simulink model "RTPS_2018a"  (R2018a)
settings: Solver=FixedStepAuto  StartTime=0.0  StopTime=150  RelTol=1e-3
settings Model: Creator=root  LastModifiedBy=bzhan
settings RTWCC: Description=Create Visual C/C++ Solution File for Simulink Coder  TemplateMakefile=RTW.MSVCBuild
settings CodeAppCC: StateflowObjectComments=on

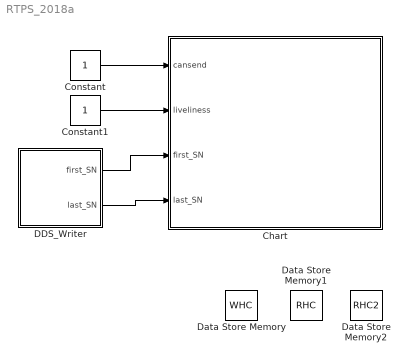
== system RTPS_2018a ==
  Chart : Stateflow chart  TreatAsAtomicUnit=on
  Constant : Constant
  Constant1 : Constant
  DDS_Writer : Stateflow chart  TreatAsAtomicUnit=on
  Data Store Memory : DataStoreMemory  DataStoreName=WHC  ReadBeforeWriteMsg=warning  WriteAfterWriteMsg=warning  WriteAfterReadMsg=warning  InitialValue=[0 0 0 0 0]  ShowAdditionalParam=off  OutDataTypeStr=int32
  Data Store Memory1 : DataStoreMemory  DataStoreName=RHC  ReadBeforeWriteMsg=warning  WriteAfterWriteMsg=warning  WriteAfterReadMsg=warning  InitialValue=[0 0 0 0 0]  VectorParams1D=off  ShowAdditionalParam=off  OutDataTypeStr=int32
  Data Store Memory2 : DataStoreMemory  DataStoreName=RHC2  ReadBeforeWriteMsg=warning  WriteAfterWriteMsg=warning  WriteAfterReadMsg=warning  InitialValue=[0 0 0 0 0]  VectorParams1D=off  ShowAdditionalParam=off  OutDataTypeStr=int32
  wires:
  Constant/1 -> Chart/1(cansend)
  Constant1/1 -> Chart/2(liveliness)
  DDS_Writer/1(first_SN) -> Chart/3(first_SN)
  DDS_Writer/2(last_SN) -> Chart/4(last_SN)

== stateflow chart RTPS_2018a/DDS_Writer ==
  state add
  (default) -> add : {i=1;first_SN=1;last_SN=0;d=random()}
  add -> add : after(d,sec)[i<=5]
      | {WHC(i)=cachechanges(i);
      | first_SN=1;last_SN=i;i = i + 1;d=random()}
  data: y function_output; i local; first_SN output; last_SN output; WHC data_store_memory; flag local; cachechanges local =[100,200,300,400,500]; d local
  function y=random:
    | function y=random
    |   y=rand();

== stateflow chart RTPS_2018a/Chart ==
  state select_channel(i) [function]
    (junction 462) -> (junction 468) [order 1] : [i==1]
    (junction 468) -> (junction 471) : {send(TRY,model.channel.channel_1)}
    (junction 462) -> (junction 466) [order 2] : [i==2]
    (junction 466) -> (junction 471) : {send(TRY,model.channel.channel_2)}
    (default) -> (junction 462)
    (junction 462) -> (junction 465) [order 3] : [i==3]
    (junction 465) -> (junction 471) : {send(TRY,model.channel.channel_3)}
    (junction 462) -> (junction 464) [order 4] : [i==4]
    (junction 462) -> (junction 463) [order 5]
    (junction 464) -> (junction 471) : {send(TRY,model.channel.channel_4)}
    (junction 463) -> (junction 471) : {send(TRY,model.channel.channel_5)}
  state set_acknack(wid,rid,rn,mn) [function]
    (default) -> (junction 110)
    (junction 110) -> (junction 103) : {buffer_acknack(rid,1)=1;
        | buffer_acknack(rid,2)=rid}
    (junction 103) -> (junction 104) : {buffer_acknack(rid,3)=rn;
        | buffer_acknack(rid,4)=mn}
  state flag=acked_all [function]
    (junction 625) -> (junction 624) [order 3]
    (junction 624) -> (junction 627) : {flag=0}
    (default) -> (junction 625) : {i=1}
    (junction 625) -> (junction 626) [order 1] : [i>2]
    (junction 626) -> (junction 627) : {flag=1}
    (junction 627) -> (junction 628)
    (junction 630) -> (junction 625)
    (junction 625) -> (junction 631) [order 2] : [i<=2&&buffer_acknack(i,3)==5]
    (junction 631) -> (junction 630) : {i = i + 1}
  state flag=empty [function]
    (junction 11) -> (junction 10) [order 3]
    (junction 10) -> (junction 13) : {flag=0}
    (default) -> (junction 11) : {i=first_SN}
    (junction 11) -> (junction 12) [order 1] : [i>last_SN]
    (junction 12) -> (junction 13) : {flag=1}
    (junction 13) -> (junction 14)
    (junction 16) -> (junction 11)
    (junction 11) -> (junction 18) [order 2] : [i<=last_SN&&unsent(i)==0]
    (junction 18) -> (junction 16) : {i = i + 1}
  state count1 = set_final_Flag(wid,count) [function]
    (junction 33) -> (junction 34) [order 2] : {buffer_heartbeat(wid,1)=SET;count1 = count + 1}
    (junction 34) -> (junction 35)
    (default) -> (junction 33)
    (junction 33) -> (junction 36) [order 1] : [count==3]
    (junction 37) -> (junction 34)
    (junction 36) -> (junction 37) : {buffer_heartbeat(wid,1)=NO_SET;count1=0}
  state set_liveliness_Flag(wid, flag) [function]
    (default) -> (junction 27)
    (junction 27) -> (junction 48) : {buffer_heartbeat(wid,2)=flag;}
  state set_heartbeatSN(wid) [function]
    (default) -> (junction 79)
    (junction 79) -> (junction 80) : {buffer_heartbeat(wid,3)=first_SN}
    (junction 80) -> (junction 81) : {buffer_heartbeat(wid,4)=last_SN}
  state set_message(sn) [function]
    (junction 606) -> (junction 83) : {buffer_data(WriterId,i,sn)=WHC(sn);i = i + 1}
    (junction 83) -> (junction 47)
    (junction 47) -> (junction 606) [order 1] : [i<=2]
    (default) -> (junction 47) : {i=1}
    (junction 47) -> (junction 611) [order 2]
  state model
    state RTPS_Reader [parallel]
      settings: executionOrder=2
      state RTPS_Reader_2 [parallel]
        settings: executionOrder=2
        state Reader_receive [parallel]
          settings: executionOrder=1
          state ready
          model.RTPS_Reader.RTPS_Reader_2.Reader_receive.ready -> model.RTPS_Reader.RTPS_Reader_2.Reader_receive.ready [order 2] : SUCCESS[seq_num_2>received_num2]
              | {index2=seq_num_2;
              | received_set(ReaderId_2,index2)=true;
              | received_num2=check_received(WriterId,ReaderId_2,received_num2);
              | missing_num2=check_missing(WriterId,ReaderId_2,missing_num2);
              | RHC2(index2)=buffer_data(WriterId,ReaderId_2,index2);
              | buffer_data(WriterId,ReaderId_2,index2)=false}
          model.RTPS_Reader.RTPS_Reader_2.Reader_receive.ready -> model.RTPS_Reader.RTPS_Reader_2.Reader_receive.ready [order 1] : HEARTBEAT2
              | {missing_num2=get_heartbeatSN(1,2);}
          (default) -> model.RTPS_Reader.RTPS_Reader_2.Reader_receive.ready
        state Reader_response [parallel]
          settings: executionOrder=2
          state must_send_ack
          state may_send_ack
          state waiting
          model.RTPS_Reader.RTPS_Reader_2.Reader_response.must_send_ack -> model.RTPS_Reader.RTPS_Reader_2.Reader_response.waiting : after(nackResponseDelay,sec)
              | {ack_id=ReaderId_2;
              | set_acknack(WriterId,ack_id,received_num2,missing_num2);
              | send(ACKNACK,model.channel_Acknack_2);
              | hFlag=0}
          model.RTPS_Reader.RTPS_Reader_2.Reader_response.may_send_ack -> model.RTPS_Reader.RTPS_Reader_2.Reader_response.must_send_ack [order 1] : [missing_num2>received_num2]
          (junction 191) -> model.RTPS_Reader.RTPS_Reader_2.Reader_response.must_send_ack [order 1] : [buffer_heartbeat(WriterId, livelinessFlag)==NO_SET]
          model.RTPS_Reader.RTPS_Reader_2.Reader_response.waiting -> (junction 191) : HEARTBEAT2{hFlag=1}
          (default) -> model.RTPS_Reader.RTPS_Reader_2.Reader_response.waiting
          (junction 191) -> model.RTPS_Reader.RTPS_Reader_2.Reader_response.may_send_ack [order 3]
          (junction 191) -> model.RTPS_Reader.RTPS_Reader_2.Reader_response.waiting [order 2] : [buffer_heartbeat(WriterId, finalFlag)==SET]{hFlag=0}
          model.RTPS_Reader.RTPS_Reader_2.Reader_response.may_send_ack -> model.RTPS_Reader.RTPS_Reader_2.Reader_response.waiting [order 2] : [missing_num2<=received_num2]{hFlag=0}
      state RTPS_Reader_1 [parallel]
        settings: executionOrder=1
        state Reader_receive [parallel]
          settings: executionOrder=1
          state ready
          model.RTPS_Reader.RTPS_Reader_1.Reader_receive.ready -> model.RTPS_Reader.RTPS_Reader_1.Reader_receive.ready [order 2] : SUCCESS[seq_num_1>received_num]
              | {index=seq_num_1;received_set(WriterId,index)=true;
              | received_num=check_received(WriterId,ReaderId_1,received_num);
              | missing_num=check_missing(WriterId,ReaderId_1,missing_num);
              | RHC(index)=buffer_data(WriterId,ReaderId_1,index);
              | buffer_data(WriterId,ReaderId_1,index)=false;}
          (default) -> model.RTPS_Reader.RTPS_Reader_1.Reader_receive.ready
          model.RTPS_Reader.RTPS_Reader_1.Reader_receive.ready -> model.RTPS_Reader.RTPS_Reader_1.Reader_receive.ready [order 1] : HEARTBEAT2
              | {missing_num=get_heartbeatSN(1,1);}
        state Reader_response [parallel]
          settings: executionOrder=2
          state must_send_ack
          state waiting
          state may_send_ack
          model.RTPS_Reader.RTPS_Reader_1.Reader_response.must_send_ack -> model.RTPS_Reader.RTPS_Reader_1.Reader_response.waiting : after(nackResponseDelay,sec)
              | {ack_id=ReaderId_1;
              | set_acknack(WriterId,ack_id,received_num,missing_num);
              | send(ACKNACK,model.channel_Acknack_1);
              | hFlag=0}
          model.RTPS_Reader.RTPS_Reader_1.Reader_response.may_send_ack -> model.RTPS_Reader.RTPS_Reader_1.Reader_response.must_send_ack [order 1] : [missing_num>received_num]
          (junction 224) -> model.RTPS_Reader.RTPS_Reader_1.Reader_response.must_send_ack [order 1] : [buffer_heartbeat(WriterId, livelinessFlag)==NO_SET]
          model.RTPS_Reader.RTPS_Reader_1.Reader_response.waiting -> (junction 224) : HEARTBEAT2{hFlag=1}
          (junction 224) -> model.RTPS_Reader.RTPS_Reader_1.Reader_response.may_send_ack [order 3]
          (junction 224) -> model.RTPS_Reader.RTPS_Reader_1.Reader_response.waiting [order 2] : [buffer_heartbeat(WriterId, finalFlag)==SET]
              | {hFlag=0}
          (default) -> model.RTPS_Reader.RTPS_Reader_1.Reader_response.waiting
          model.RTPS_Reader.RTPS_Reader_1.Reader_response.may_send_ack -> model.RTPS_Reader.RTPS_Reader_1.Reader_response.waiting [order 2] : [missing_num<=received_num]{hFlag=0}
    state RTPS_Writer [parallel]
      settings: executionOrder=1
      state Writer_send [parallel]
        settings: executionOrder=2
        state pushing
        state announcing
        state idle
        announcing -> (junction 771) [order 1] : after(heartbeatPeriod,sec)
            | [acked_all()==false&&empty()==true]
            | {hb_count=set_final_Flag(WriterId,hb_count);
            | set_liveliness_Flag(WriterId, liveliness);
            | set_heartbeatSN(WriterId);
            | send(HEARTBEAT,model.channel_Heartbeat);
            |  sendFlag=1}
        (junction 771) -> announcing : {sendFlag=0}
        pushing -> pushing [order 2] : [cansend==true&&empty()==false]
            | {set_message(index);
            | select_channel(index);
            | unsent(index) = false;
            | index = index + 1}
        idle -> announcing : [acked_all()==false]
        announcing -> pushing [order 2] : [acked_all()==false&&empty()==false]
        announcing -> idle [order 3] : [acked_all()==true]{complete=true}
        pushing -> announcing [order 1] : [empty()==true]
        (default) -> announcing : {init()}
      state Writer_repair [parallel]
        settings: executionOrder=1
        state repairing
        state waiting
        state must_repair
          state en
          (default) -> en : {ackFlag=0}
          en -> en : ACKNACK2{id=ack_id;
              |  [acked_num(id),request_num(id)]=get_acknack(WriterId,id);
              | ackFlag=1}
        repairing -> repairing [order 1] : [cansend==true&&repair_num(id)<=request_num(id)]
            | {set_message(repair_num(id));
            | select_channel(repair_num(id));
            | repair_num(id) = repair_num(id) + 1}
        must_repair -> repairing : after(heartbeatResponseDelay,sec)
            | {repair_num(id)=acked_num(id)+1;
            | ackFlag=0}
        repairing -> model.RTPS_Writer.Writer_repair.waiting [order 2] : [cansend==false||repair_num(id)>request_num(id)]
        model.RTPS_Writer.Writer_repair.waiting -> must_repair [order 1] : [id>0&&request_num(id)>acked_num(id)]
        (default) -> model.RTPS_Writer.Writer_repair.waiting
        model.RTPS_Writer.Writer_repair.waiting -> model.RTPS_Writer.Writer_repair.waiting [order 2] : ACKNACK2
            | [id<=0||request_num(id)<=acked_num(id)]
            | {id=ack_id;
            | [acked_num(id),request_num(id)]=get_acknack(WriterId,id);
            | ackFlag=1}
    state channel_Heartbeat [parallel]
      settings: executionOrder=4
      state try
      state delay
      (default) -> model.channel_Heartbeat.try
      (junction 764) -> model.channel_Heartbeat.try [order 2]
      model.channel_Heartbeat.try -> (junction 764) : HEARTBEAT
      model.channel_Heartbeat.delay -> model.channel_Heartbeat.try : after(d_hb,sec)
          | {send(HEARTBEAT2,model.RTPS_Reader)}
      (junction 764) -> model.channel_Heartbeat.delay [order 1] : [channel()==true]{d_hb=delay()}
    state channel_Acknack_1 [parallel]
      settings: executionOrder=5
      state try
      state delay
      (default) -> model.channel_Acknack_1.try
      (junction 723) -> model.channel_Acknack_1.try [order 2]
      model.channel_Acknack_1.try -> (junction 723) : ACKNACK
      model.channel_Acknack_1.delay -> model.channel_Acknack_1.try : after(d_ack1,sec)
          | {ack_id=ReaderId_1;
          | send(ACKNACK2,model.RTPS_Writer)}
      (junction 723) -> model.channel_Acknack_1.delay [order 1] : [channel()==true]{d_ack1=delay()}
    state channel [parallel]
      settings: executionOrder=3
      state channel_4 [parallel]
        settings: executionOrder=4
        state try
        state delay_1
        state delay_2
        state next
        (default) -> model.channel.channel_4.try
        model.channel.channel_4.next -> model.channel.channel_4.try [order 2] : {buffer_data(WriterId,2,4)=0}
        model.channel.channel_4.try -> (junction 553) : TRY
        model.channel.channel_4.delay_2 -> model.channel.channel_4.try : after(d4,sec)
            | {seq_num_2=4;
            | send(SUCCESS,model.RTPS_Reader.RTPS_Reader_2)}
        (junction 553) -> model.channel.channel_4.delay_1 [order 1] : [channel()==true]{d4=delay()}
        (junction 553) -> model.channel.channel_4.next [order 2] : {buffer_data(WriterId,1,4)=0}
        model.channel.channel_4.delay_1 -> model.channel.channel_4.next : after(d4,sec)
            | {seq_num_1=4;
            | send(SUCCESS,model.RTPS_Reader.RTPS_Reader_1)}
        model.channel.channel_4.next -> model.channel.channel_4.delay_2 [order 1] : [channel()==true]{d4=delay()}
      state channel_5 [parallel]
        settings: executionOrder=5
        state try
        state delay_1
        state delay_2
        state next
        (default) -> model.channel.channel_5.try
        model.channel.channel_5.next -> model.channel.channel_5.try [order 2] : {buffer_data(WriterId,2,5)=0}
        model.channel.channel_5.try -> (junction 571) : TRY
        model.channel.channel_5.delay_2 -> model.channel.channel_5.try : after(d5,sec)
            | {seq_num_2=5;
            | send(SUCCESS,model.RTPS_Reader.RTPS_Reader_2)}
        (junction 571) -> model.channel.channel_5.delay_1 [order 1] : [channel()==true]{d5=delay()}
        (junction 571) -> model.channel.channel_5.next [order 2] : {buffer_data(WriterId,1,5)=0}
        model.channel.channel_5.delay_1 -> model.channel.channel_5.next : after(d5,sec)
            | {seq_num_1=5;
            | send(SUCCESS,model.RTPS_Reader.RTPS_Reader_1)}
        model.channel.channel_5.next -> model.channel.channel_5.delay_2 [order 1] : [channel()==true]{d5=delay()}
      state channel_2 [parallel]
        settings: executionOrder=2
        state try
        state delay_1
        state delay_2
        state next
        (default) -> model.channel.channel_2.try
        model.channel.channel_2.next -> model.channel.channel_2.try [order 2] : {buffer_data(WriterId,2,2)=0}
        model.channel.channel_2.try -> (junction 517) : TRY
        model.channel.channel_2.delay_2 -> model.channel.channel_2.try : after(d2,sec)
            | {seq_num_2=2;
            | send(SUCCESS,model.RTPS_Reader.RTPS_Reader_2)}
        (junction 517) -> model.channel.channel_2.delay_1 [order 1] : [channel()==true]{d2=delay()}
        (junction 517) -> model.channel.channel_2.next [order 2] : {buffer_data(WriterId,1,2)=0}
        model.channel.channel_2.delay_1 -> model.channel.channel_2.next : after(d2,sec)
            | {seq_num_1=2;
            | send(SUCCESS,model.RTPS_Reader.RTPS_Reader_1)}
        model.channel.channel_2.next -> model.channel.channel_2.delay_2 [order 1] : [channel()==true]{d2=delay()}
      state channel_3 [parallel]
        settings: executionOrder=3
        state try
        state delay_1
        state delay_2
        state next
        (default) -> model.channel.channel_3.try
        model.channel.channel_3.next -> model.channel.channel_3.try [order 2] : {buffer_data(WriterId,2,3)=0}
        model.channel.channel_3.try -> (junction 535) : TRY
        model.channel.channel_3.delay_2 -> model.channel.channel_3.try : after(d3,sec)
            | {seq_num_2=3;
            | send(SUCCESS,model.RTPS_Reader.RTPS_Reader_2)}
        (junction 535) -> model.channel.channel_3.delay_1 [order 1] : [channel()==true]{d3=delay()}
        (junction 535) -> model.channel.channel_3.next [order 2] : {buffer_data(WriterId,1,3)=0}
        model.channel.channel_3.delay_1 -> model.channel.channel_3.next : after(d3,sec)
            | {seq_num_1=3;
            | send(SUCCESS,model.RTPS_Reader.RTPS_Reader_1)}
        model.channel.channel_3.next -> model.channel.channel_3.delay_2 [order 1] : [channel()==true]{d3=delay()}
      state channel_1 [parallel]
        settings: executionOrder=1
        state try
        state delay_1
        state delay_2
        state next
        model.channel.channel_1.next -> model.channel.channel_1.try [order 2] : {buffer_data(WriterId,ReaderId_1,1)=0}
        (default) -> model.channel.channel_1.try
        model.channel.channel_1.try -> (junction 360) : TRY
        model.channel.channel_1.delay_2 -> model.channel.channel_1.try : after(d1,sec)
            | {seq_num_2=1;
            | send(SUCCESS,model.RTPS_Reader.RTPS_Reader_2)}
        (junction 360) -> model.channel.channel_1.delay_1 [order 1] : [channel()==true]{d1=delay()}
        (junction 360) -> model.channel.channel_1.next [order 2] : {buffer_data(WriterId,ReaderId_2,1)=0}
        model.channel.channel_1.delay_1 -> model.channel.channel_1.next : after(d1,sec)
            | {seq_num_1=1;
            | send(SUCCESS,model.RTPS_Reader.RTPS_Reader_1)}
        model.channel.channel_1.next -> model.channel.channel_1.delay_2 [order 1] : [channel()==true]{d1=delay()}
    state channel_Acknack_2 [parallel]
      settings: executionOrder=6
      state try
      state delay
      (default) -> model.channel_Acknack_2.try
      (junction 807) -> model.channel_Acknack_2.try [order 2]
      model.channel_Acknack_2.try -> (junction 807) : ACKNACK
      model.channel_Acknack_2.delay -> model.channel_Acknack_2.try : after(d_ack2,sec)
          | {ack_id=ReaderId_2;
          | send(ACKNACK2,model.RTPS_Writer)}
      (junction 807) -> model.channel_Acknack_2.delay [order 1] : [channel()==true]{d_ack2=delay()}
  state [an,rn]=get_acknack(wid,rid) [function]
    (default) -> (junction 90)
    (junction 90) -> (junction 91) : {an=buffer_acknack(rid,3)}
    (junction 91) -> (junction 92) : {rn=buffer_acknack(rid,4)}
  state sn2  = check_missing(wid, rid,sn1) [function]
    (junction 123) -> (junction 121) [order 2] : {sn2=i}
    (default) -> (junction 122)
    (junction 122) -> (junction 123) : {i=sn1}
    (junction 125) -> (junction 123)
    (junction 123) -> (junction 124) [order 1] : [i>=1&&received_set(rid,i)==true]
    (junction 124) -> (junction 125) : {i = i -1}
  state sn2  = check_received(wid, rid,sn1) [function]
    (default) -> (junction 150) : {i=sn1+1}
    (junction 150) -> (junction 151) [order 2] : {sn2=i-1}
    (junction 153) -> (junction 150)
    (junction 150) -> (junction 152) [order 1] : [i<=5&&received_set(rid,i)==true]
    (junction 152) -> (junction 153) : {i = i + 1}
  state lastSN=get_heartbeatSN(wid,rid) [function]
    (default) -> (junction 146)
    (junction 146) -> (junction 145) : {firstSN=buffer_heartbeat(wid,3);
        | lastSN=buffer_heartbeat(wid,4)}
  (default) -> model
  data: i function_input; wid function_input; rid function_input; rn function_input; mn function_input; flag function_output; flag function_output; y function_output; wid function_input; count function_input; count1 function_output; wid function_input; flag function_input; wid function_input; sn function_input; hFlag local =0; index2 local =0; received_num2 local =0; missing_num2 local =0; hFlag local =0; index local =0; received_num local =0; missing_num local =0; hb_count local =0; sendFlag local =0; ackFlag local =0; index local =1; repair_num local size=[1 2] =[0 0]; id local =0; request_num local size=[1 2] =[0 0]; id local; id local; id local; id local; id local; id local; id local; id local; wid function_input; rid function_input; an function_output; rn function_output; chan_r function_output; wid function_input; sn2 function_output; rid function_input; sn1 function_input; wid function_input; sn2 function_output; rid function_input; sn1 function_input; wid function_input; rid function_input; lastSN function_output; cansend input; liveliness input; buffer_heartbeat local size=[1 4] =[[0 0 0 0]]; unsent local size=[1 5] =[1 1 1 1 1]; RHC data_store_memory; buffer_acknack local size=[2 4] =[0 0 0 0 ; 0 0 0 0]; WHC data_store_memory; RHC2 data_store_memory; ack_id local =0; received_set local size=[2 5] =[0 0 0 0 0;0 0 0 0 0]; buffer_data local size=[1 2 5]; seq_num_1 local =0; seq_num_2 local =0; SET constant int32 =0; NO_SET constant double =1; nackResponseDelay constant double =1; heartbeatResponseDelay constant double =1.5; heartbeatPeriod constant double =1.5; first_SN input; last_SN input; data local; data1 local; acked_num local size=[1 2] =[0 0]; WriterId local =1; finalFlag local =2; livelinessFlag local =1; ReaderId_1 local =1; ReaderId_2 local =2; d1 local; d2 local; d3 local; d4 local; d5 local; d_ack1 local; d_ack2 local; d_hb local
  events: HEARTBEAT local FUNCTION_CALL_EVENT; ACKNACK local FUNCTION_CALL_EVENT; TRY local FUNCTION_CALL_EVENT; SUCCESS local FUNCTION_CALL_EVENT; SUCCESS2 local FUNCTION_CALL_EVENT; ACKNACK2 local FUNCTION_CALL_EVENT; HEARTBEAT2 local FUNCTION_CALL_EVENT
  function y=delay:
    | function y=delay
    |   y=rand();
  function chan_r=channel:
    | function chan_r=channel()
    |   x=rand();
    |   if x>0.4
    |       chan_r=1;
    |   else
    |       chan_r=0; 
    |   end
  function init:
    | function init
    |   buffer_data=zeros(1,2,5);
    |   end
